simulink library "lib_lowphy"  (R2023b)
settings: Solver=VariableStepAuto  StartTime=0.0  StopTime=10.0  RelTol=1e-3
undefined symbols (not defined in the file or in its folder): AdvDSPBChannelOutDisplay, AdvDSPBDMemDisplay, AdvDSPBInDisplay, AdvDSPBOutDisplay, dpoly, dspba, dspba_ChannelInVis, dspba_ChannelOutVis, dspba_internal_get_channel_ports, evalAionMaskParam, fft_tb_in, ifft_tb_in, latency, latencyCorrection, max_FFTStages, max_NSubcarriers, primtype, UseDontCare, value
libraries: DSPBAPrim x637, DSPBAControl x55, $bdroot x16, DSPBAModelBus x12, DSPBAUtilities x6, DSPBABase x5, DSPBAWaveformSynth x4, DspbAdvFftLibrary x3, DSPBAVectorUtil x2, DspbAdvVfftPrefix x1
(part 3 of 9)

== system lib_lowphy/PhaseCompensation_lite/SOP_EOP_gen ==
  vin : Inport
  chin : Inport  Port=2
  din : Inport  Port=3
  eAxC_in : Inport  Port=4
  And : DSPBAPrim/And  primtype=and  nInputs=2  nOutputs=1  omode=Inherit via internal rule  otype=sfix(16)  scale=2^-15  rndmethod=Unbiased  factor=1  satmethod=Symmetric  shift_vec=[0 1 2 -1]  value=0  inPortNames=[' '; ' '; ' '; ' '; ' '; ' '; ' '; ' '; ' '; ' '; ' '; ' '; ' '; ' '; ' '; ' '; ]  outPortNames=[' ']  dspbaimage=dspba_prim.svg  text=fprintf('&');  style=Optimised  visibilities=8+2  version=20211007
  And1 : DSPBAPrim/And  primtype=and  nInputs=2  nOutputs=1  omode=Inherit via internal rule  otype=sfix(16)  scale=2^-15  rndmethod=Unbiased  factor=1  satmethod=Symmetric  shift_vec=[0 1 2 -1]  value=0  inPortNames=[' '; ' '; ' '; ' '; ' '; ' '; ' '; ' '; ' '; ' '; ' '; ' '; ' '; ' '; ' '; ' '; ]  outPortNames=[' ']  dspbaimage=dspba_prim.svg  text=fprintf('&');  style=Optimised  visibilities=8+2  version=20211007
  CmpEQ : DSPBAPrim/CmpEQ  primtype=cmpeq  nInputs=2  nOutputs=1  omode=boolean  otype=sfix(16)  scale=2^-15  rndmethod=Unbiased  factor=1  satmethod=Symmetric  shift_vec=[0 1 2 -1]  value=0  inPortNames=[' '; ' ';]  outPortNames=[' ']  dspbaimage=dspba_prim.svg  text=fprintf('==');  style=Optimised  visibilities=0  advOptions=[]  version=20211007
  CmpEQ1 : DSPBAPrim/CmpEQ  primtype=cmpeq  nInputs=2  nOutputs=1  omode=boolean  otype=sfix(16)  scale=2^-15  rndmethod=Unbiased  factor=1  satmethod=Symmetric  shift_vec=[0 1 2 -1]  value=0  inPortNames=[' '; ' ';]  outPortNames=[' ']  dspbaimage=dspba_prim.svg  text=fprintf('==');  style=Optimised  visibilities=0  advOptions=[]  version=20211007
  Const : DSPBAPrim/Const  primtype=const  nInputs=0  nOutputs=1  omode=Specify via dialog  otype=uint(8)  scale=2^0  rndmethod=Unbiased  factor=1  satmethod=Symmetric  shift_vec=[0 1 2 -1]  value=3  inPortNames=['+'; '+';]  outPortNames=[' ']  dspbaimage=dspba_prim.svg  text=fprintf('%s', num2str(value));  style=Optimised  visibilities=8 + 1024  floatPrecision=float32_m23  warnSaturation=on  version=20211007  SampleTime=inf
  Const1 : DSPBAPrim/Const  primtype=const  nInputs=0  nOutputs=1  omode=Specify via dialog  otype=uint(8)  scale=2^0  rndmethod=Unbiased  factor=1  satmethod=Symmetric  shift_vec=[0 1 2 -1]  value=0  inPortNames=['+'; '+';]  outPortNames=[' ']  dspbaimage=dspba_prim.svg  text=fprintf('%s', num2str(value));  style=Optimised  visibilities=8 + 1024  floatPrecision=float32_m23  warnSaturation=on  version=20211007  SampleTime=inf
  Rising_edge : Subsystem
      mask init:
      | fsmpaths
  SampleDelay{1..4} (4 alike) : DSPBAPrim/SampleDelay  primtype=sampdelay  nInputs=1  nOutputs=1  omode=Inherit via internal rule  otype=sfix(16)  scale=2^-15  rndmethod=Unbiased  factor=1  satmethod=Symmetric  shift_vec=[0 1 2 -1]  floatPrecision=float32_m23  value=1  inPortNames=[' '; ' ';]  outPortNames=[' ']  dspbaimage=dspba_prim.svg  text=dpoly(1, eye(1,value+1), 'z')  style=Optimised  visibilities=8 + 1024 + 2^17 + 2^18  flexible=off  slackgroup=0  augmented=3  version=20211007  advOptions=[]
  SynthesisInfo : DSPBAPrim/SynthesisInfo  primtype=synthinfo  nInputs=0  nOutputs=0  omode=Inherit via internal rule  otype=sfix(16)  scale=2^-15  rndmethod=Truncate  factor=1  satmethod=Symmetric  shift_vec=[0 1 2 -1]  value=99  inPortNames=[' '; ' ';]  outPortNames=[' ']  dspbaimage=dspba_prim_ctrl.jpg  text=fprintf('Style=%s', style);  style=Scheduled  visibilities=2^17+2^18+2^19+2^20+2^21+2^22+2^23+2^24  constraintPair=None  constraintRelation=>  constraintLimit=2  modelRefSign=+  modelRef=''  showSchedule=off  simulationMode=Use Global Value  resetMinimization=Conditional - On for ChannelIn/Out only  version=20220106
  channel_RXG1_in : DSPBAPrim/ChannelIn  primtype=channelin  nInputs=dspba_internal_get_channel_ports(gcb)  nOutputs=dspba_internal_get_channel_ports(gcb)  omode=Inherit via internal rule  otype=sfix(16)  scale=2^-15  rndmethod=Unbiased  factor=1  satmethod=Symmetric  shift_vec=[0 1 2 -1]  value=2  inPortNames=['v'; 'c'; '0'; '1'; '2'; '3'; '4'; '5'; '6'; '7'; '8'; '9'; 'A'; 'B'; 'D'; 'E'; 'F'; 'G'; 'H'; 'I'; 'J'; 'K'; 'L'; 'M'; 'N'; 'O'; 'P'; 'Q'; 'R'; 'S'; 'T'; 'U'; 'W'; 'X'; 'Y'; 'Z']  outPortNames=['v'; 'c'; '0'; '1'; '2'; '3'; '4'; '5'; '6'; '7'; '8'; '9'; 'A'; 'B'; 'D'; 'E'; 'F'; 'G'; 'H'; 'I'; 'J'; 'K'; 'L'; 'M'; 'N'; 'O'; 'P'; 'Q'; 'R'; 'S'; 'T'; 'U'; 'W'; 'X'; 'Y'; 'Z']  dspbaimage=dspba_prim_channel_tall.svg  text=fprintf('In');  style=Optimised  dataSignals=2  foldingEnabled=off  channels=1  sampleRate=200  packetBeginPresent=off  packetBeginEnabled=off  visibilities=dspba_ChannelInVis(gcb)  latencyCorrection=0  scheduleOrigin=on  version=20211214
  channel_RXG1_out : DSPBAPrim/ChannelOut  primtype=channelout  nInputs=dspba_internal_get_channel_ports(gcb)  nOutputs=dspba_internal_get_channel_ports(gcb)  omode=Inherit via internal rule  otype=sfix(16)  scale=2^-15  rndmethod=Unbiased  factor=1  satmethod=Symmetric  shift_vec=[0 1 2 -1]  value=6  inPortNames=['v'; 'c'; '0'; '1'; '2'; '3'; '4'; '5'; '6'; '7'; '8'; '9'; 'A'; 'B'; 'D'; 'E'; 'F'; 'G'; 'H'; 'I'; 'J'; 'K'; 'L'; 'M'; 'N'; 'O'; 'P'; 'Q'; 'R'; 'S'; 'T'; 'U'; 'W'; 'X'; 'Y'; 'Z']  outPortNames=['v'; 'c'; '0'; '1'; '2'; '3'; '4'; '5'; '6'; '7'; '8'; '9'; 'A'; 'B'; 'D'; 'E'; 'F'; 'G'; 'H'; 'I'; 'J'; 'K'; 'L'; 'M'; 'N'; 'O'; 'P'; 'Q'; 'R'; 'S'; 'T'; 'U'; 'W'; 'X'; 'Y'; 'Z']  dspbaimage=dspba_prim_channel_tall.svg  text=fprintf('Out%s', AdvDSPBChannelOutDisplay(latency));  style=Optimised  dataSignals=6  foldingEnabled=off  channels=1  sampleRate=200  packetBeginPresent=off  packetBeginEnabled=off  visibilities=dspba_ChannelOutVis(gcb)  latency=8  latencyCorrection=0  version=20211214
  falling_edge : Subsystem
      mask init:
      | fsmpaths
  vout : Outport
  chout : Outport  Port=2
  dout : Outport  Port=3
  eAxC_out : Outport  Port=4
  eop_eAxC : Outport  Port=5
  eop_sym : Outport  Port=6
  sop_eAxC : Outport  Port=7
  sop_sym : Outport  Port=8
  wires:
  falling_edge/1(falling_edge) -> And/1, channel_RXG1_out/5
  channel_RXG1_out/4 -> eAxC_out/1
  channel_RXG1_in/1 -> falling_edge/1(in), SampleDelay2/1
  channel_RXG1_in/4 -> CmpEQ/2, SampleDelay4/1
  channel_RXG1_out/1 -> vout/1
  channel_RXG1_out/5 -> eop_eAxC/1
  channel_RXG1_out/6 -> eop_sym/1
  vin/1 -> channel_RXG1_in/1
  channel_RXG1_in/2 -> SampleDelay1/1
  eAxC_in/1 -> channel_RXG1_in/4
  chin/1 -> channel_RXG1_in/2
  din/1 -> channel_RXG1_in/3
  channel_RXG1_in/3 -> SampleDelay3/1
  channel_RXG1_out/2 -> chout/1
  Const/1 -> CmpEQ/1
  And/1 -> channel_RXG1_out/6
  channel_RXG1_out/3 -> dout/1
  CmpEQ/1 -> And/2
  SampleDelay2/1 -> Rising_edge/1(in), channel_RXG1_out/1
  SampleDelay1/1 -> channel_RXG1_out/2
  SampleDelay3/1 -> channel_RXG1_out/3
  channel_RXG1_out/7 -> sop_eAxC/1
  channel_RXG1_out/8 -> sop_sym/1
  Const1/1 -> CmpEQ1/1
  SampleDelay4/1 -> CmpEQ1/2, channel_RXG1_out/4
  Rising_edge/1(rising_edge) -> And1/1, channel_RXG1_out/7
  CmpEQ1/1 -> And1/2
  And1/1 -> channel_RXG1_out/8

== system lib_lowphy/iFFT_B2S/B2S ==
  v_in : Inport
  c_in : Inport  Port=2
  q_in : Inport  Port=3
  sizein : Inport  Port=4
  cplen : Inport  Port=5
  nprb : Inport  Port=6
  B2S_Inst : Subsystem
  vout1 : Outport
  cout1 : Outport  Port=2
  dout1 : Outport  Port=3
  wires:
  cplen/1 -> B2S_Inst/5(cplen)
  c_in/1 -> B2S_Inst/2(chin)
  q_in/1 -> B2S_Inst/3(din)
  sizein/1 -> B2S_Inst/4(FFTSize)
  v_in/1 -> B2S_Inst/1(vin)
  B2S_Inst/1(vout) -> vout1/1
  B2S_Inst/2(cout) -> cout1/1
  B2S_Inst/3(q) -> dout1/1
  nprb/1 -> B2S_Inst/6(nprb)

== system lib_lowphy/iFFT_B2S/IFFT ==
  note: VIFFT :4 AxCs of 100 MHz
  data1 : Inport
  valid1 : Inport  Port=2
  channel1 : Inport  Port=3
  size1 : Inport  Port=4
  cplen1 : Inport  Port=5
  nsc1 : Inport  Port=6
  ifft_gain_re_l1 : Inport  Port=7
  ifft_gain_im_l1 : Inport  Port=8
  ifft_shift_l1 : Inport  Port=9
  ifft_mux_const_l1 : Inport  Port=10
  muxsel_l1 : Inport  Port=11
  DC_SC_EN : Inport  Port=12
  ripple_comp_en : Inport  Port=13
  rc_bw_sel : Inport  Port=14
  time_in : Inport  Port=15
  Input_signal_latch : Subsystem
  VIFFT : Subsystem
  vout1 : Outport
  cout1 : Outport  Port=2
  dout1 : Outport  Port=3
  sizeout1 : Outport  Port=4
  cpout1 : Outport  Port=5
  nprb : Outport  Port=6
  fd_data_v : Outport  Port=7
  fd_data_c : Outport  Port=8
  fd_data_q : Outport  Port=9
  fd_time_out : Outport  Port=10
  wires:
  VIFFT/1(dout) -> dout1/1
  VIFFT/5(cplen_Out) -> cpout1/1
  VIFFT/3(cout) -> cout1/1
  valid1/1 -> Input_signal_latch/1(valid)
  Input_signal_latch/5(q_nprb) -> VIFFT/6(nsc)
  Input_signal_latch/2(qchannel) -> VIFFT/3(channel)
  ifft_mux_const_l1/1 -> Input_signal_latch/11(ifft_mux_const_data)
  VIFFT/2(vout) -> vout1/1
  Input_signal_latch/4(qfftsize) -> VIFFT/4(size)
  Input_signal_latch/9(qf_ift_gain_imag) -> VIFFT/8(ifft_gain_im)
  cplen1/1 -> Input_signal_latch/6(cplen)
  data1/1 -> Input_signal_latch/3(data)
  Input_signal_latch/6(qcplen) -> VIFFT/5(cplen)
  Input_signal_latch/7(q_dc_sc_en) -> VIFFT/12(DC_SC_EN)
  Input_signal_latch/3(qdata) -> VIFFT/1(data)
  ifft_gain_im_l1/1 -> Input_signal_latch/9(ifftgain_imag)
  Input_signal_latch/11(q_ifft_mux_const_data) -> VIFFT/10(ifft_mux_const)
  VIFFT/4(sizeout) -> sizeout1/1
  Input_signal_latch/10(q_ifftshift) -> VIFFT/9(ifft_shift)
  Input_signal_latch/12(q_muxsel) -> VIFFT/11(muxsel)
  Input_signal_latch/8(qfft_gain_real) -> VIFFT/7(ifft_gain_re)
  Input_signal_latch/1(qvalid) -> VIFFT/2(valid)
  DC_SC_EN/1 -> Input_signal_latch/7(DC_SC_EN1)
  nsc1/1 -> Input_signal_latch/5(NSubCarr)
  muxsel_l1/1 -> Input_signal_latch/12(muxsel)
  ifft_shift_l1/1 -> Input_signal_latch/10(ifftshift)
  ifft_gain_re_l1/1 -> Input_signal_latch/8(iftgain_real)
  size1/1 -> Input_signal_latch/4(FFTSize)
  channel1/1 -> Input_signal_latch/2(ch)
  VIFFT/6(nprb) -> nprb/1
  ripple_comp_en/1 -> VIFFT/13(ripple_comp_en)
  rc_bw_sel/1 -> VIFFT/14(rc_bw_sel)
  VIFFT/7(fd_data_v) -> fd_data_v/1
  VIFFT/8(fd_data_c) -> fd_data_c/1
  VIFFT/9(fd_data_q) -> fd_data_q/1
  time_in/1 -> Input_signal_latch/13(time_in)
  Input_signal_latch/13(time_out) -> VIFFT/15(time_in)
  VIFFT/10(fd_time_out) -> fd_time_out/1

== system lib_lowphy/FFT_S2B/CPRemoval/Incr_Symbol_out_val ==
  dv : Inport
  Sym_counter_meta_data : Subsystem
  Sym_out_meta : Outport
  wires:
  Sym_counter_meta_data/1(Sym_out_meta) -> Sym_out_meta/1
  dv/1 -> Sym_counter_meta_data/1(Data_write_valid)

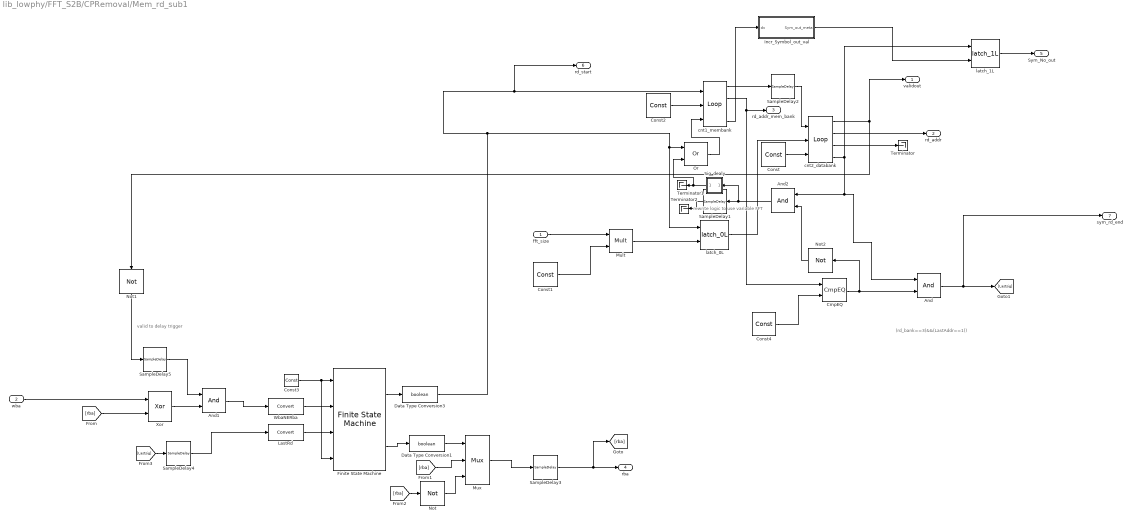
== system lib_lowphy/FFT_S2B/CPRemoval/Mem_rd_sub1 ==
  note: rewrite logic to use variable FFT
  note: (rd_bank==3)&&(LastAddr==1))
  note: valid to delay trigger
  fft_size : Inport
  wba : Inport  Port=2
  And : DSPBAPrim/And  primtype=and  nInputs=2  nOutputs=1  omode=Inherit via internal rule  otype=sfix(16)  scale=2^-15  rndmethod=Unbiased  factor=1  satmethod=Symmetric  shift_vec=[0 1 2 -1]  value=0  inPortNames=[' '; ' '; ' '; ' '; ' '; ' '; ' '; ' '; ' '; ' '; ' '; ' '; ' '; ' '; ' '; ' '; ]  outPortNames=[' ']  dspbaimage=dspba_prim.svg  text=fprintf('&');  style=Optimised  visibilities=8+2  version=20211007
  And1 : DSPBAPrim/And  primtype=and  nInputs=2  nOutputs=1  omode=Inherit via internal rule  otype=sfix(16)  scale=2^-15  rndmethod=Unbiased  factor=1  satmethod=Symmetric  shift_vec=[0 1 2 -1]  value=0  inPortNames=[' '; ' '; ' '; ' '; ' '; ' '; ' '; ' '; ' '; ' '; ' '; ' '; ' '; ' '; ' '; ' '; ]  outPortNames=[' ']  dspbaimage=dspba_prim.svg  text=fprintf('&');  style=Optimised  visibilities=8+2  version=20211007
  And2 : DSPBAPrim/And  primtype=and  nInputs=2  nOutputs=1  omode=Inherit via internal rule  otype=sfix(16)  scale=2^-15  rndmethod=Unbiased  factor=1  satmethod=Symmetric  shift_vec=[0 1 2 -1]  value=0  inPortNames=[' '; ' '; ' '; ' '; ' '; ' '; ' '; ' '; ' '; ' '; ' '; ' '; ' '; ' '; ' '; ' '; ]  outPortNames=[' ']  dspbaimage=dspba_prim.svg  text=fprintf('&');  style=Optimised  visibilities=8+2  version=20211007
  CmpEQ : DSPBAPrim/CmpEQ  primtype=cmpeq  nInputs=2  nOutputs=1  omode=boolean  otype=sfix(16)  scale=2^-15  rndmethod=Unbiased  factor=1  satmethod=Symmetric  shift_vec=[0 1 2 -1]  value=0  inPortNames=[' '; ' ';]  outPortNames=[' ']  dspbaimage=dspba_prim.svg  text=fprintf('==');  style=Optimised  visibilities=0  advOptions=[]  version=20211007
  Const : DSPBAPrim/Const  primtype=const  nInputs=0  nOutputs=1  omode=boolean  otype=sfix(16)  scale=2^-15  rndmethod=Unbiased  factor=1  satmethod=Symmetric  shift_vec=[0 1 2 -1]  value=1  inPortNames=['+'; '+';]  outPortNames=[' ']  dspbaimage=dspba_prim.svg  text=fprintf('%s', num2str(value));  style=Optimised  visibilities=8 + 1024  floatPrecision=float32_m23  warnSaturation=on  version=20211007  SampleTime=inf
  Const1 : DSPBAPrim/Const  primtype=const  nInputs=0  nOutputs=1  omode=Specify via dialog  otype=fixdt(0,3,0)  scale=0  rndmethod=Unbiased  factor=1  satmethod=Symmetric  shift_vec=[0 1 2 -1]  value=1  inPortNames=['+'; '+';]  outPortNames=[' ']  dspbaimage=dspba_prim.svg  text=fprintf('%s', num2str(value));  style=Optimised  visibilities=8 + 1024  floatPrecision=float32_m23  warnSaturation=on  version=20211007  SampleTime=inf
  Const2 : DSPBAPrim/Const  primtype=const  nInputs=0  nOutputs=1  omode=Specify via dialog  otype=fixdt(0,3,0)  scale=0  rndmethod=Unbiased  factor=1  satmethod=Symmetric  shift_vec=[0 1 2 -1]  value=4  inPortNames=['+'; '+';]  outPortNames=[' ']  dspbaimage=dspba_prim.svg  text=fprintf('%s', num2str(value));  style=Optimised  visibilities=8 + 1024  floatPrecision=float32_m23  warnSaturation=on  version=20211007  SampleTime=inf
  Const3 : DSPBAPrim/Const  primtype=const  nInputs=0  nOutputs=1  omode=Specify via dialog  otype=ufix(1)  scale=1  rndmethod=Unbiased  factor=1  satmethod=Symmetric  shift_vec=[0 1 2 -1]  value=1  inPortNames=['+'; '+';]  outPortNames=[' ']  dspbaimage=dspba_prim.svg  text=fprintf('%s', num2str(value));  style=Optimised  visibilities=8 + 1024  floatPrecision=float32_m23  warnSaturation=on  version=20211007  SampleTime=inf
  Const4 : DSPBAPrim/Const  primtype=const  nInputs=0  nOutputs=1  omode=Specify via dialog  otype=fixdt(0,3,0)  scale=0  rndmethod=Unbiased  factor=1  satmethod=Symmetric  shift_vec=[0 1 2 -1]  value=3  inPortNames=['+'; '+';]  outPortNames=[' ']  dspbaimage=dspba_prim.svg  text=fprintf('%s', num2str(value));  style=Optimised  visibilities=8 + 1024  floatPrecision=float32_m23  warnSaturation=on  version=20211007  SampleTime=inf
  Data Type Conversion1 : DataTypeConversion  OutDataTypeStr=boolean  SaturateOnIntegerOverflow=off  RndMeth=Floor
  Data Type Conversion3 : DataTypeConversion  OutDataTypeStr=boolean  SaturateOnIntegerOverflow=off  RndMeth=Floor
  Finite State Machine : DSPBAUtilities/Finite State Machine  desc_file=demo_fsm_control_read_s2b.fsm  latency=0  simulationMode=Bit And Cycle Accurate  finiteStateMachine=on
  Incr_Symbol_out_val : Subsystem
  LastRd : DataTypeConversion  SaturateOnIntegerOverflow=off  RndMeth=Floor
  Mult : DSPBAPrim/Mult  primtype=mult  nInputs=2  nOutputs=1  omode=Inherit via internal rule  otype=sfix(16)  scale=2^-15  rndmethod=Unbiased  factor=1  satmethod=Symmetric  shift_vec=[0 1 2 -1]  value=0  inPortNames=[' '; ' ';]  outPortNames=[' ']  dspbaimage=dspba_prim.svg  text=fprintf('X');  style=Optimised  visibilities=8+2^18+2^19  floatPrecision=float32_m23  floatRounding=correct  advOptions=[]  version=20211007
  Mux : DSPBAPrim/Mux  primtype=mux  nInputs=evalAionMaskParam(gcb,'value',1)+1  nOutputs=1  omode=Inherit via internal rule  otype=sfix(16)  scale=2^-15  rndmethod=Unbiased  factor=1  satmethod=Symmetric  shift_vec=[0 1 2 -1]  value=2  inPortNames=['s '; 'd0'; 'd1'; 'd2'; 'd3'; 'd4'; 'd5'; 'd6'; 'd7'; 'd8'; 'd9';]  outPortNames=[' ']  dspbaimage=dspba_prim_tall.svg  text=fprintf('%s', primtype);  style=Optimised  visibilities=1032  version=20211007
  Not : DSPBAPrim/Not  primtype=not  nInputs=1  nOutputs=1  omode=Inherit via internal rule  otype=sfix(16)  scale=2^-15  rndmethod=Unbiased  factor=1  satmethod=Symmetric  shift_vec=[0 1 2 -1]  value=0  inPortNames=[' '; ' ';]  outPortNames=[' ']  dspbaimage=dspba_prim.svg  text=fprintf('~');  style=Optimised  visibilities=8  version=20211007
  Not1 : DSPBAPrim/Not  primtype=not  nInputs=1  nOutputs=1  omode=Inherit via internal rule  otype=sfix(16)  scale=2^-15  rndmethod=Unbiased  factor=1  satmethod=Symmetric  shift_vec=[0 1 2 -1]  value=0  inPortNames=[' '; ' ';]  outPortNames=[' ']  dspbaimage=dspba_prim.svg  text=fprintf('~');  style=Optimised  visibilities=8  version=20211007
  Not2 : DSPBAPrim/Not  primtype=not  nInputs=1  nOutputs=1  omode=Inherit via internal rule  otype=sfix(16)  scale=2^-15  rndmethod=Unbiased  factor=1  satmethod=Symmetric  shift_vec=[0 1 2 -1]  value=0  inPortNames=[' '; ' ';]  outPortNames=[' ']  dspbaimage=dspba_prim.svg  text=fprintf('~');  style=Optimised  visibilities=8  version=20211007
  Or : DSPBAPrim/Or  primtype=or  nInputs=2  nOutputs=1  omode=Inherit via internal rule  otype=sfix(16)  scale=2^-15  rndmethod=Unbiased  factor=1  satmethod=Symmetric  shift_vec=[0 1 2 -1]  value=0  inPortNames=[' '; ' '; ' '; ' '; ' '; ' '; ' '; ' '; ' '; ' '; ' '; ' '; ' '; ' '; ' '; ' '; ]  outPortNames=[' ']  dspbaimage=dspba_prim.svg  text=fprintf('|');  style=Optimised  visibilities=8+2  version=20211007
  SampleDelay1 : DSPBAPrim/SampleDelay  primtype=sampdelay  nInputs=1  nOutputs=1  omode=Inherit via internal rule  otype=sfix(16)  scale=2^-15  rndmethod=Unbiased  factor=1  satmethod=Symmetric  shift_vec=[0 1 2 -1]  floatPrecision=float32_m23  value=288  inPortNames=[' '; ' ';]  outPortNames=[' ']  dspbaimage=dspba_prim.svg  text=dpoly(1, eye(1,value+1), 'z')  style=Optimised  visibilities=8 + 1024 + 2^17 + 2^18  flexible=off  slackgroup=0  augmented=0  version=20211007  advOptions=[]
  SampleDelay2 : DSPBAPrim/SampleDelay  primtype=sampdelay  nInputs=1  nOutputs=1  omode=Inherit via internal rule  otype=sfix(16)  scale=2^-15  rndmethod=Unbiased  factor=1  satmethod=Symmetric  shift_vec=[0 1 2 -1]  floatPrecision=float32_m23  value=1  inPortNames=[' '; ' ';]  outPortNames=[' ']  dspbaimage=dspba_prim.svg  text=dpoly(1, eye(1,value+1), 'z')  style=Optimised  visibilities=8 + 1024 + 2^17 + 2^18  flexible=on  slackgroup=0  augmented=3  version=20211007  advOptions=[]
  SampleDelay3 : DSPBAPrim/SampleDelay  primtype=sampdelay  nInputs=1  nOutputs=1  omode=boolean  otype=sfix(16)  scale=2^-15  rndmethod=Unbiased  factor=1  satmethod=Symmetric  shift_vec=[0 1 2 -1]  floatPrecision=float32_m23  value=1  inPortNames=[' '; ' ';]  outPortNames=[' ']  dspbaimage=dspba_prim.svg  text=dpoly(1, eye(1,value+1), 'z')  style=Optimised  visibilities=8 + 1024 + 2^17 + 2^18  flexible=off  slackgroup=0  augmented=0  version=20211007  advOptions=[]
  SampleDelay4 : DSPBAPrim/SampleDelay  primtype=sampdelay  nInputs=1  nOutputs=1  omode=Inherit via internal rule  otype=sfix(16)  scale=2^-15  rndmethod=Unbiased  factor=1  satmethod=Symmetric  shift_vec=[0 1 2 -1]  floatPrecision=float32_m23  value=1  inPortNames=[' '; ' ';]  outPortNames=[' ']  dspbaimage=dspba_prim.svg  text=dpoly(1, eye(1,value+1), 'z')  style=Optimised  visibilities=8 + 1024 + 2^17 + 2^18  flexible=off  slackgroup=0  augmented=0  version=20211007  advOptions=[]
  SampleDelay5 : DSPBAPrim/SampleDelay  primtype=sampdelay  nInputs=1  nOutputs=1  omode=Inherit via internal rule  otype=sfix(16)  scale=2^-15  rndmethod=Unbiased  factor=1  satmethod=Symmetric  shift_vec=[0 1 2 -1]  floatPrecision=float32_m23  value=10  inPortNames=[' '; ' ';]  outPortNames=[' ']  dspbaimage=dspba_prim.svg  text=dpoly(1, eye(1,value+1), 'z')  style=Optimised  visibilities=8 + 1024 + 2^17 + 2^18  flexible=off  slackgroup=0  augmented=0  version=20211007  advOptions=[]
  Sig_dealy : Subsystem
  Terminator : Terminator
  Terminator1 : Terminator
  Terminator2 : Terminator
  WbaNERba : DataTypeConversion  SaturateOnIntegerOverflow=off  RndMeth=Floor
  Xor : DSPBAPrim/Xor  primtype=xor  nInputs=2  nOutputs=1  omode=boolean  otype=sfix(16)  scale=2^-15  rndmethod=Unbiased  factor=1  satmethod=Symmetric  shift_vec=[0 1 2 -1]  value=0  inPortNames=[' '; ' '; ' '; ' '; ' '; ' '; ' '; ' '; ' '; ' '; ' '; ' '; ' '; ' '; ' '; ' '; ]  outPortNames=[' ']  dspbaimage=dspba_prim.svg  text=fprintf('^');  style=Optimised  visibilities=8+2  version=20211007
  cnt1_membank : DSPBAPrim/Loop  primtype=loop  nInputs=3  nOutputs=4  omode=Inherit via internal rule  otype=sfix(16)  scale=2^-15  rndmethod=Unbiased  factor=1  satmethod=Symmetric  shift_vec=[0 1 2 -1]  value=[zeros(16, 1)]  inPortNames=['g'; 'c'; 'e']  outPortNames=['v'; 'q'; 'f'; 'l']  dspbaimage=dspba_prim_tall.svg  text=fprintf('loop');  style=Optimised  visibilities=0  version=20211007
  cnt2_databank : DSPBAPrim/Loop  primtype=loop  nInputs=3  nOutputs=4  omode=Inherit via internal rule  otype=sfix(16)  scale=2^-15  rndmethod=Unbiased  factor=1  satmethod=Symmetric  shift_vec=[0 1 2 -1]  value=[zeros(16, 1)]  inPortNames=['g'; 'c'; 'e']  outPortNames=['v'; 'q'; 'f'; 'l']  dspbaimage=dspba_prim_tall.svg  text=fprintf('loop');  style=Optimised  visibilities=0  version=20211007
  latch_0L : DSPBAControl/latch_0L
  latch_1L : DSPBAControl/latch_1L
  validout : Outport
  rd_addr : Outport  Port=2
  rd_addr_mem_bank : Outport  Port=3
  rba : Outport  Port=4
  Sym_No_out : Outport  Port=5
  rd_start : Outport  Port=6
  sym_rd_end : Outport  Port=7
  wires:
  cnt2_databank/2 -> rd_addr/1
  cnt2_databank/1 -> validout/1, Not1/1
  cnt2_databank/3 -> Terminator/1
  Data Type Conversion3/1 -> rd_start/1, cnt1_membank/1, latch_0L/1, Or/1
  latch_0L/1 -> cnt2_databank/2
  Const/1 -> cnt2_databank/3
  Mult/1 -> latch_0L/2
  fft_size/1 -> Mult/1
  Const1/1 -> Mult/2
  Const2/1 -> cnt1_membank/2
  cnt1_membank/1 -> SampleDelay2/1
  cnt1_membank/2 -> CmpEQ/1, rd_addr_mem_bank/1
  SampleDelay2/1 -> cnt2_databank/1
  Or/1 -> cnt1_membank/3
  Const3/1 -> Finite State Machine/4, Finite State Machine/1
  [Lastsig] -> SampleDelay4/1
  Finite State Machine/1 -> Data Type Conversion3/1
  LastRd/1 -> Finite State Machine/3
  WbaNERba/1 -> Finite State Machine/2
  wba/1 -> Xor/1
  SampleDelay3/1 -> [rba], rba/1
  Mux/1 -> SampleDelay3/1
  [rba] -> Xor/2
  [rba] -> Mux/2
  Not/1 -> Mux/3
  [rba] -> Not/1
  Const4/1 -> CmpEQ/2
  CmpEQ/1 -> And/2, Not2/1
  And/1 -> sym_rd_end/1, [Lastsig]
  SampleDelay4/1 -> LastRd/1
  Data Type Conversion1/1 -> Mux/1
  Finite State Machine/2 -> Data Type Conversion1/1
  And1/1 -> WbaNERba/1
  Xor/1 -> And1/2
  SampleDelay5/1 -> And1/1
  Not1/1 -> SampleDelay5/1
  cnt2_databank/4 -> latch_1L/1, And2/1, And/1
  And2/1 -> Sig_dealy/1(In1), SampleDelay1/1
  Not2/1 -> And2/2
  Sig_dealy/1(Out1) -> Or/2, Terminator1/1
  cnt1_membank/4 -> Incr_Symbol_out_val/1(dv)
  latch_1L/1 -> Sym_No_out/1
  Incr_Symbol_out_val/1(Sym_out_meta) -> latch_1L/2
  SampleDelay1/1 -> Terminator2/1

== system lib_lowphy/FFT_S2B/CPRemoval/Mem_wr_subsystem ==
  valid : Inport
  CPlen : Inport  Port=2
  FFTlen : Inport  Port=3
  NumAxc : Inport  Port=4
  Const : DSPBAPrim/Const  primtype=const  nInputs=0  nOutputs=1  omode=boolean  otype=sfix(16)  scale=2^-15  rndmethod=Unbiased  factor=1  satmethod=Symmetric  shift_vec=[0 1 2 -1]  value=1  inPortNames=['+'; '+';]  outPortNames=[' ']  dspbaimage=dspba_prim.svg  text=fprintf('%s', num2str(value));  style=Optimised  visibilities=8 + 1024  floatPrecision=float32_m23  warnSaturation=on  version=20211007  SampleTime=inf
  Const1 : DSPBAPrim/Const  primtype=const  nInputs=0  nOutputs=1  omode=boolean  otype=sfix(16)  scale=2^-15  rndmethod=Unbiased  factor=1  satmethod=Symmetric  shift_vec=[0 1 2 -1]  value=1  inPortNames=['+'; '+';]  outPortNames=[' ']  dspbaimage=dspba_prim.svg  text=fprintf('%s', num2str(value));  style=Optimised  visibilities=8 + 1024  floatPrecision=float32_m23  warnSaturation=on  version=20211007  SampleTime=inf
  Const2 : DSPBAPrim/Const  primtype=const  nInputs=0  nOutputs=1  omode=Specify via dialog  otype=ufix(1)  scale=1  rndmethod=Unbiased  factor=1  satmethod=Symmetric  shift_vec=[0 1 2 -1]  value=1  inPortNames=['+'; '+';]  outPortNames=[' ']  dspbaimage=dspba_prim.svg  text=fprintf('%s', num2str(value));  style=Optimised  visibilities=8 + 1024  floatPrecision=float32_m23  warnSaturation=on  version=20211007  SampleTime=inf
  Data Type Conversion : DataTypeConversion  SaturateOnIntegerOverflow=off  RndMeth=Floor
  Data Type Conversion1 : DataTypeConversion  OutDataTypeStr=boolean  SaturateOnIntegerOverflow=off  RndMeth=Floor
  Data Type Conversion2 : DataTypeConversion  OutDataTypeStr=boolean  SaturateOnIntegerOverflow=off  RndMeth=Floor
  Data Type Conversion3 : DataTypeConversion  OutDataTypeStr=boolean  SaturateOnIntegerOverflow=off  RndMeth=Floor
  Finite State Machine : DSPBAUtilities/Finite State Machine  desc_file=demo_fsm_control.fsm  latency=0  simulationMode=Bit And Cycle Accurate  finiteStateMachine=on
  LShift : DSPBAPrim/LShift  primtype=lshift  nInputs=2  nOutputs=1  omode=Specify via dialog  otype=fixdt(0,12,0)  scale=0  rndmethod=Unbiased  factor=1  satmethod=Symmetric  shift_vec=[0 1 2 -1]  value=0  inPortNames=['a'; 'b';]  outPortNames=[' ']  dspbaimage=dspba_prim.svg  text=fprintf('a << b');  style=Optimised  visibilities=8  version=20211007
  LShift1 : DSPBAPrim/LShift  primtype=lshift  nInputs=2  nOutputs=1  omode=Specify via dialog  otype=fixdt(0,17,0)  scale=0  rndmethod=Unbiased  factor=1  satmethod=Symmetric  shift_vec=[0 1 2 -1]  value=0  inPortNames=['a'; 'b';]  outPortNames=[' ']  dspbaimage=dspba_prim.svg  text=fprintf('a << b');  style=Optimised  visibilities=8  version=20211007
  Lastsig_gen : Subsystem
  Lastsig_gen1 : $bdroot/FFT_S2B/CPRemoval/Mem_wr_subsystem/Lastsig_gen  SystemSampleTime=-1  VariantActivationTime=update diagram  AllowFlexibleInterface=on  Latency=0  AutoFrameSizeCalculation=off
  Mux : DSPBAPrim/Mux  primtype=mux  nInputs=evalAionMaskParam(gcb,'value',1)+1  nOutputs=1  omode=Inherit via internal rule  otype=sfix(16)  scale=2^-15  rndmethod=Unbiased  factor=1  satmethod=Symmetric  shift_vec=[0 1 2 -1]  value=2  inPortNames=['s '; 'd0'; 'd1'; 'd2'; 'd3'; 'd4'; 'd5'; 'd6'; 'd7'; 'd8'; 'd9';]  outPortNames=[' ']  dspbaimage=dspba_prim_tall.svg  text=fprintf('%s', primtype);  style=Optimised  visibilities=1032  version=20211007
  Not : DSPBAPrim/Not  primtype=not  nInputs=1  nOutputs=1  omode=Inherit via internal rule  otype=sfix(16)  scale=2^-15  rndmethod=Unbiased  factor=1  satmethod=Symmetric  shift_vec=[0 1 2 -1]  value=0  inPortNames=[' '; ' ';]  outPortNames=[' ']  dspbaimage=dspba_prim.svg  text=fprintf('~');  style=Optimised  visibilities=8  version=20211007
  SampleDelay3 : DSPBAPrim/SampleDelay  primtype=sampdelay  nInputs=1  nOutputs=1  omode=boolean  otype=sfix(16)  scale=2^-15  rndmethod=Unbiased  factor=1  satmethod=Symmetric  shift_vec=[0 1 2 -1]  floatPrecision=float32_m23  value=1  inPortNames=[' '; ' ';]  outPortNames=[' ']  dspbaimage=dspba_prim.svg  text=dpoly(1, eye(1,value+1), 'z')  style=Optimised  visibilities=8 + 1024 + 2^17 + 2^18  flexible=off  slackgroup=0  augmented=0  version=20211007  advOptions=[]
  Terminator{,1..5} (6 alike) : Terminator
  cmp1in : DataTypeConversion  SaturateOnIntegerOverflow=off  RndMeth=Floor
  cmpin2 : DataTypeConversion  SaturateOnIntegerOverflow=off  RndMeth=Floor
  cnt1_cpcnt : DSPBAPrim/Loop  primtype=loop  nInputs=3  nOutputs=4  omode=Inherit via internal rule  otype=sfix(16)  scale=2^-15  rndmethod=Unbiased  factor=1  satmethod=Symmetric  shift_vec=[0 1 2 -1]  value=[zeros(16, 1)]  inPortNames=['g'; 'c'; 'e']  outPortNames=['v'; 'q'; 'f'; 'l']  dspbaimage=dspba_prim_tall.svg  text=fprintf('loop');  style=Optimised  visibilities=0  version=20211007
  cnt2_datalen : DSPBAPrim/Loop  primtype=loop  nInputs=3  nOutputs=4  omode=Inherit via internal rule  otype=sfix(16)  scale=2^-15  rndmethod=Unbiased  factor=1  satmethod=Symmetric  shift_vec=[0 1 2 -1]  value=[zeros(16, 1)]  inPortNames=['g'; 'c'; 'e']  outPortNames=['v'; 'q'; 'f'; 'l']  dspbaimage=dspba_prim_tall.svg  text=fprintf('loop');  style=Optimised  visibilities=0  version=20211007
  latch_0L : DSPBAControl/latch_0L
  latch_0L1 : DSPBAControl/latch_0L
  validout : Outport
  Wr_addr : Outport  Port=2
  wba : Outport  Port=3
  sym_wr_start : Outport  Port=4
  wires:
  Lastsig_gen1/1 -> Mux/1, cmpin2/1
  Const2/1 -> Finite State Machine/5, Finite State Machine/1
  Data Type Conversion3/1 -> latch_0L1/1, latch_0L/1
  SampleDelay3/1 -> Mux/2, Not/1, wba/1
  latch_0L/1 -> LShift/1
  Data Type Conversion2/1 -> Lastsig_gen1/2, cnt2_datalen/1
  Const/1 -> cnt1_cpcnt/3
  cnt1_cpcnt/3 -> Terminator3/1
  cnt2_datalen/1 -> Lastsig_gen1/4, validout/1
  LShift1/1 -> Lastsig_gen1/1, cnt2_datalen/2
  NumAxc/1 -> LShift/2, LShift1/2
  cmpin2/1 -> Finite State Machine/4
  CPlen/1 -> latch_0L/2
  LShift/1 -> Lastsig_gen/1(CountMax), cnt1_cpcnt/2
  cnt2_datalen/2 -> Lastsig_gen1/3, Wr_addr/1
  cnt1_cpcnt/2 -> Lastsig_gen/3(Runningcnt), Terminator2/1
  FFTlen/1 -> latch_0L1/2
  Finite State Machine/1 -> Data Type Conversion3/1
  Data Type Conversion/1 -> Finite State Machine/2
  Finite State Machine/3 -> Data Type Conversion1/1
  Finite State Machine/5 -> Terminator5/1
  Mux/1 -> SampleDelay3/1
  Not/1 -> Mux/3
  cmp1in/1 -> Finite State Machine/3
  Finite State Machine/2 -> Terminator4/1
  cnt1_cpcnt/1 -> Lastsig_gen/4(valid), Terminator1/1
  cnt2_datalen/3 -> Terminator/1
  Finite State Machine/4 -> Data Type Conversion2/1
  latch_0L1/1 -> LShift1/1
  Const1/1 -> cnt2_datalen/3
  Data Type Conversion1/1 -> Lastsig_gen/2(latch), cnt1_cpcnt/1
  valid/1 -> Data Type Conversion/1
  Lastsig_gen/1(Lastsig) -> cmp1in/1
  cnt1_cpcnt/4 -> sym_wr_start/1

== system lib_lowphy/FFT_S2B/CPRemoval/Nprb_fifo ==
  qv : Inport
  v : Inport  Port=2
  d : Inport  Port=3
  FIFO : DSPBAPrim/FIFO  primtype=fifo  nInputs=3  nOutputs=4  omode=Inherit via internal rule  otype=sfix(16)  scale=2^-15  rndmethod=Unbiased  factor=1  satmethod=Symmetric  shift_vec=[0 1 2 -1]  value=[16 16 16]  inPortNames=['w'; 'd'; 'r'; 'f']  outPortNames=['v'; 'q'; 't'; 'f']  dspbaimage=dspba_prim_tall.svg  text=fprintf('fifo');  style=Optimised  visibilities=263168  version=20211007  user_sclr=off
  RISING_EDGE1 : Subsystem
  RISING_EDGE3 : Subsystem
  Terminator1 : Terminator
  Terminator2 : Terminator
  Terminator3 : Terminator
  latch_0L3 : DSPBAControl/latch_0L
  q : Outport
  wires:
  FIFO/2 -> latch_0L3/2
  RISING_EDGE3/1(q) -> latch_0L3/1, FIFO/3
  FIFO/3 -> Terminator2/1
  latch_0L3/1 -> q/1
  d/1 -> FIFO/2
  FIFO/4 -> Terminator3/1
  v/1 -> RISING_EDGE1/1(d)
  qv/1 -> RISING_EDGE3/1(d)
  FIFO/1 -> Terminator1/1
  RISING_EDGE1/1(q) -> FIFO/1

== system lib_lowphy/FFT_S2B/CPRemoval/cp_len ==
  cplen : Inport
  sym_det : Inport  Port=2
  fftsize : Inport  Port=3
  CmpEQ : DSPBAPrim/CmpEQ  primtype=cmpeq  nInputs=2  nOutputs=1  omode=boolean  otype=sfix(16)  scale=2^-15  rndmethod=Unbiased  factor=1  satmethod=Symmetric  shift_vec=[0 1 2 -1]  value=0  inPortNames=[' '; ' ';]  outPortNames=[' ']  dspbaimage=dspba_prim.svg  text=fprintf('==');  style=Optimised  visibilities=0  advOptions=[]  version=20211007
  CmpEQ1 : DSPBAPrim/CmpEQ  primtype=cmpeq  nInputs=2  nOutputs=1  omode=boolean  otype=sfix(16)  scale=2^-15  rndmethod=Unbiased  factor=1  satmethod=Symmetric  shift_vec=[0 1 2 -1]  value=0  inPortNames=[' '; ' ';]  outPortNames=[' ']  dspbaimage=dspba_prim.svg  text=fprintf('==');  style=Optimised  visibilities=0  advOptions=[]  version=20211007
  Const1 : DSPBAPrim/Const  primtype=const  nInputs=0  nOutputs=1  omode=Inherit via internal rule  otype=sfix(16)  scale=2^-15  rndmethod=Unbiased  factor=1  satmethod=Symmetric  shift_vec=[0 1 2 -1]  value=0.9  inPortNames=['+'; '+';]  outPortNames=[' ']  dspbaimage=dspba_prim.svg  text=fprintf('%s', num2str(value));  style=Optimised  visibilities=8 + 1024  floatPrecision=float32_m23  warnSaturation=on  version=20211007  SampleTime=inf
  Const12 : DSPBAPrim/Const  primtype=const  nInputs=0  nOutputs=1  omode=Inherit via internal rule  otype=sfix(16)  scale=2^-15  rndmethod=Unbiased  factor=1  satmethod=Symmetric  shift_vec=[0 1 2 -1]  value=0.8181  inPortNames=['+'; '+';]  outPortNames=[' ']  dspbaimage=dspba_prim.svg  text=fprintf('%s', num2str(value));  style=Optimised  visibilities=8 + 1024  floatPrecision=float32_m23  warnSaturation=on  version=20211007  SampleTime=inf
  Const2 : DSPBAPrim/Const  primtype=const  nInputs=0  nOutputs=1  omode=Inherit via internal rule  otype=sfix(16)  scale=2^-15  rndmethod=Unbiased  factor=1  satmethod=Symmetric  shift_vec=[0 1 2 -1]  value=0  inPortNames=['+'; '+';]  outPortNames=[' ']  dspbaimage=dspba_prim.svg  text=fprintf('%s', num2str(value));  style=Optimised  visibilities=8 + 1024  floatPrecision=float32_m23  warnSaturation=on  version=20211007  SampleTime=inf
  Const3 : DSPBAPrim/Const  primtype=const  nInputs=0  nOutputs=1  omode=Inherit via internal rule  otype=sfix(16)  scale=2^-15  rndmethod=Unbiased  factor=1  satmethod=Symmetric  shift_vec=[0 1 2 -1]  value=12  inPortNames=['+'; '+';]  outPortNames=[' ']  dspbaimage=dspba_prim.svg  text=fprintf('%s', num2str(value));  style=Optimised  visibilities=8 + 1024  floatPrecision=float32_m23  warnSaturation=on  version=20211007  SampleTime=inf
  Convert : DSPBAPrim/Convert  primtype=convert  nInputs=1  nOutputs=1  omode=Specify via dialog  otype=ufix(11)  scale=2^-0  rndmethod=Biased  factor=1  satmethod=None  shift_vec=[0 1 2 -1]  value=round([0:255]/17)  inPortNames=[' '; ' ';]  outPortNames=[' '; 'c']  dspbaimage=dspba_prim_wide.svg  text=fprintf('convert');  style=Optimised  visibilities=8+64+256+2^17  clipdetect=off  floatPrecision=float32_m23  advOptions=[]  version=20211007
  Mult : DSPBAPrim/Mult  primtype=mult  nInputs=2  nOutputs=1  omode=Inherit via internal rule  otype=sfix(16)  scale=2^-15  rndmethod=Unbiased  factor=1  satmethod=Symmetric  shift_vec=[0 1 2 -1]  value=0  inPortNames=[' '; ' ';]  outPortNames=[' ']  dspbaimage=dspba_prim.svg  text=fprintf('X');  style=Optimised  visibilities=8+2^18+2^19  floatPrecision=float32_m23  floatRounding=correct  advOptions=[]  version=20211007
  Mux1 : DSPBAPrim/Mux  primtype=mux  nInputs=evalAionMaskParam(gcb,'value',1)+1  nOutputs=1  omode=Inherit via internal rule  otype=sfix(16)  scale=2^-15  rndmethod=Unbiased  factor=1  satmethod=Symmetric  shift_vec=[0 1 2 -1]  value=2  inPortNames=['s '; 'd0'; 'd1'; 'd2'; 'd3'; 'd4'; 'd5'; 'd6'; 'd7'; 'd8'; 'd9';]  outPortNames=[' ']  dspbaimage=dspba_prim_tall.svg  text=fprintf('%s', primtype);  style=Optimised  visibilities=1032  version=20211007
  Mux2 : DSPBAPrim/Mux  primtype=mux  nInputs=evalAionMaskParam(gcb,'value',1)+1  nOutputs=1  omode=Inherit via internal rule  otype=sfix(16)  scale=2^-15  rndmethod=Unbiased  factor=1  satmethod=Symmetric  shift_vec=[0 1 2 -1]  value=2  inPortNames=['s '; 'd0'; 'd1'; 'd2'; 'd3'; 'd4'; 'd5'; 'd6'; 'd7'; 'd8'; 'd9';]  outPortNames=[' ']  dspbaimage=dspba_prim_tall.svg  text=fprintf('%s', primtype);  style=Optimised  visibilities=1032  version=20211007
  cp_out : Outport
  wires:
  Convert/1 -> Mux2/2
  Mult/1 -> Convert/1
  cplen/1 -> Mult/1, Mux2/3
  Mux1/1 -> Mult/2
  Mux2/1 -> cp_out/1
  sym_det/1 -> CmpEQ/1
  CmpEQ/1 -> Mux2/1
  Const2/1 -> CmpEQ/2
  fftsize/1 -> CmpEQ1/1
  Const3/1 -> CmpEQ1/2
  Const12/1 -> Mux1/3
  CmpEQ1/1 -> Mux1/1
  Const1/1 -> Mux1/2

== system lib_lowphy/FFT_S2B/CPRemoval/fft_size_fifo ==
  qv : Inport
  v : Inport  Port=2
  d : Inport  Port=3
  FIFO : DSPBAPrim/FIFO  primtype=fifo  nInputs=3  nOutputs=4  omode=Inherit via internal rule  otype=sfix(16)  scale=2^-15  rndmethod=Unbiased  factor=1  satmethod=Symmetric  shift_vec=[0 1 2 -1]  value=[16 16 16]  inPortNames=['w'; 'd'; 'r'; 'f']  outPortNames=['v'; 'q'; 't'; 'f']  dspbaimage=dspba_prim_tall.svg  text=fprintf('fifo');  style=Optimised  visibilities=263168  version=20211007  user_sclr=off
  RISING_EDGE1 : Subsystem
  RISING_EDGE3 : Subsystem
  Terminator1 : Terminator
  Terminator2 : Terminator
  Terminator3 : Terminator
  latch_0L3 : DSPBAControl/latch_0L
  q : Outport
  wires:
  FIFO/2 -> latch_0L3/2
  RISING_EDGE3/1(q) -> latch_0L3/1, FIFO/3
  FIFO/3 -> Terminator2/1
  latch_0L3/1 -> q/1
  d/1 -> FIFO/2
  FIFO/4 -> Terminator3/1
  v/1 -> RISING_EDGE1/1(d)
  qv/1 -> RISING_EDGE3/1(d)
  FIFO/1 -> Terminator1/1
  RISING_EDGE1/1(q) -> FIFO/1

== system lib_lowphy/FFT_S2B/CPRemoval/sym_metadata_fffo ==
  qv : Inport
  v : Inport  Port=2
  d : Inport  Port=3
  FIFO : DSPBAPrim/FIFO  primtype=fifo  nInputs=3  nOutputs=4  omode=Inherit via internal rule  otype=sfix(16)  scale=2^-15  rndmethod=Unbiased  factor=1  satmethod=Symmetric  shift_vec=[0 1 2 -1]  value=[16 16 16]  inPortNames=['w'; 'd'; 'r'; 'f']  outPortNames=['v'; 'q'; 't'; 'f']  dspbaimage=dspba_prim_tall.svg  text=fprintf('fifo');  style=Optimised  visibilities=263168  version=20211007  user_sclr=off
  RISING_EDGE1 : Subsystem
  RISING_EDGE3 : Subsystem
  Terminator1 : Terminator
  Terminator2 : Terminator
  Terminator3 : Terminator
  q : Outport
  wires:
  RISING_EDGE3/1(q) -> FIFO/3
  FIFO/3 -> Terminator2/1
  FIFO/2 -> q/1
  d/1 -> FIFO/2
  FIFO/4 -> Terminator3/1
  v/1 -> RISING_EDGE1/1(d)
  qv/1 -> RISING_EDGE3/1(d)
  FIFO/1 -> Terminator1/1
  RISING_EDGE1/1(q) -> FIFO/1

== system lib_lowphy/FFT_S2B/CPRemoval/timeref_reg ==
  qv : Inport
  v : Inport  Port=2
  d : Inport  Port=3
  FIFO : DSPBAPrim/FIFO  primtype=fifo  nInputs=3  nOutputs=4  omode=Inherit via internal rule  otype=sfix(16)  scale=2^-15  rndmethod=Unbiased  factor=1  satmethod=Symmetric  shift_vec=[0 1 2 -1]  value=[16 16 16]  inPortNames=['w'; 'd'; 'r'; 'f']  outPortNames=['v'; 'q'; 't'; 'f']  dspbaimage=dspba_prim_tall.svg  text=fprintf('fifo');  style=Optimised  visibilities=263168  version=20211007  user_sclr=off
  RISING_EDGE1 : Subsystem
  RISING_EDGE3 : Subsystem
  Terminator1 : Terminator
  Terminator2 : Terminator
  Terminator3 : Terminator
  q : Outport
  wires:
  RISING_EDGE3/1(q) -> FIFO/3
  FIFO/3 -> Terminator2/1
  FIFO/2 -> q/1
  d/1 -> FIFO/2
  FIFO/4 -> Terminator3/1
  v/1 -> RISING_EDGE1/1(d)
  qv/1 -> RISING_EDGE3/1(d)
  FIFO/1 -> Terminator1/1
  RISING_EDGE1/1(q) -> FIFO/1

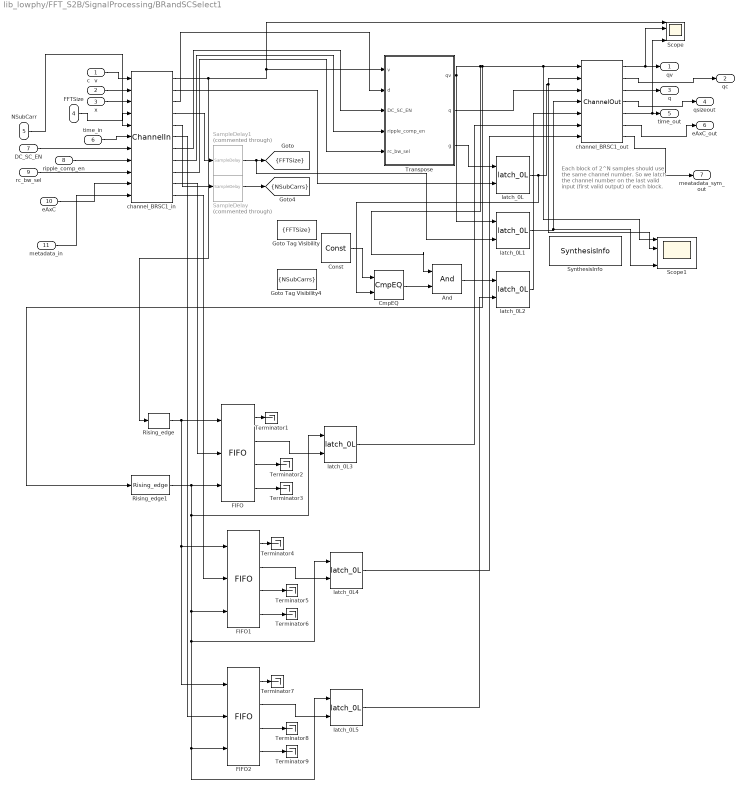
== system lib_lowphy/FFT_S2B/SignalProcessing/BRandSCSelect1 ==
  note: Each block of 2^N samples should
      |  use the same channel number.
      |
      | So we latch the channel number on
      |  the last valid input (first valid output)
      | of each block.
  v : Inport
  c : Inport  Port=2
  x : Inport  Port=3
  FFTSize : Inport  Port=4
  NSubCarr : Inport  Port=5
  time_in : Inport  Port=6
  DC_SC_EN : Inport  Port=7
  ripple_comp_en : Inport  Port=8
  rc_bw_sel : Inport  Port=9
  eAxC : Inport  Port=10
  metadata_in : Inport  Port=11
  And : DSPBAPrim/And  primtype=and  nInputs=2  nOutputs=1  omode=Inherit via internal rule  otype=sfix(16)  scale=2^-15  rndmethod=Unbiased  factor=1  satmethod=Symmetric  shift_vec=[0 1 2 -1]  value=0  inPortNames=[' '; ' '; ' '; ' '; ' '; ' '; ' '; ' '; ' '; ' '; ' '; ' '; ' '; ' '; ' '; ' '; ]  outPortNames=[' ']  dspbaimage=dspba_prim.svg  text=fprintf('&');  style=Optimised  visibilities=8+2  version=20211007
  CmpEQ : DSPBAPrim/CmpEQ  primtype=cmpeq  nInputs=2  nOutputs=1  omode=boolean  otype=sfix(16)  scale=2^-15  rndmethod=Unbiased  factor=1  satmethod=Symmetric  shift_vec=[0 1 2 -1]  value=0  inPortNames=[' '; ' ';]  outPortNames=[' ']  dspbaimage=dspba_prim.svg  text=fprintf('==');  style=Optimised  visibilities=0  advOptions=[]  version=20211007
  Const : DSPBAPrim/Const  primtype=const  nInputs=0  nOutputs=1  omode=Specify via dialog  otype=uint(8)  scale=2^0  rndmethod=Unbiased  factor=1  satmethod=Symmetric  shift_vec=[0 1 2 -1]  value=0  inPortNames=['+'; '+';]  outPortNames=[' ']  dspbaimage=dspba_prim.svg  text=fprintf('%s', num2str(value));  style=Optimised  visibilities=8 + 1024  floatPrecision=float32_m23  warnSaturation=on  version=20211007  SampleTime=inf
  FIFO : DSPBAPrim/FIFO  primtype=fifo  nInputs=3  nOutputs=4  omode=Inherit via internal rule  otype=sfix(16)  scale=2^-15  rndmethod=Unbiased  factor=1  satmethod=Symmetric  shift_vec=[0 1 2 -1]  value=[16 16 16]  inPortNames=['w'; 'd'; 'r'; 'f']  outPortNames=['v'; 'q'; 't'; 'f']  dspbaimage=dspba_prim_tall.svg  text=fprintf('fifo');  style=Optimised  visibilities=263168  version=20211007  user_sclr=off
  FIFO1 : DSPBAPrim/FIFO  primtype=fifo  nInputs=3  nOutputs=4  omode=Inherit via internal rule  otype=sfix(16)  scale=2^-15  rndmethod=Unbiased  factor=1  satmethod=Symmetric  shift_vec=[0 1 2 -1]  value=[16 16 16]  inPortNames=['w'; 'd'; 'r'; 'f']  outPortNames=['v'; 'q'; 't'; 'f']  dspbaimage=dspba_prim_tall.svg  text=fprintf('fifo');  style=Optimised  visibilities=263168  version=20211007  user_sclr=off
  FIFO2 : DSPBAPrim/FIFO  primtype=fifo  nInputs=3  nOutputs=4  omode=Inherit via internal rule  otype=sfix(16)  scale=2^-15  rndmethod=Unbiased  factor=1  satmethod=Symmetric  shift_vec=[0 1 2 -1]  value=[16 16 16]  inPortNames=['w'; 'd'; 'r'; 'f']  outPortNames=['v'; 'q'; 't'; 'f']  dspbaimage=dspba_prim_tall.svg  text=fprintf('fifo');  style=Optimised  visibilities=263168  version=20211007  user_sclr=off
  Goto Tag Visibility : GotoTagVisibility  GotoTag=FFTSize
  Goto Tag Visibility4 : GotoTagVisibility  GotoTag=NSubCarrs
  Rising_edge : $bdroot/Rising_edge
  Rising_edge1 : $bdroot/Rising_edge
  SampleDelay : DSPBAPrim/SampleDelay  Commented=through  primtype=sampdelay  nInputs=1  nOutputs=1  omode=Inherit via internal rule  otype=sfix(16)  scale=2^-15  rndmethod=Unbiased  factor=1  satmethod=Symmetric  shift_vec=[0 1 2 -1]  floatPrecision=float32_m23  value=2  inPortNames=[' '; ' ';]  outPortNames=[' ']  dspbaimage=dspba_prim.svg  text=dpoly(1, eye(1,value+1), 'z')  style=Optimised  visibilities=8 + 1024 + 2^17 + 2^18  flexible=off  slackgroup=0  augmented=0  version=20211007  advOptions=[]
  SampleDelay1 : DSPBAPrim/SampleDelay  Commented=through  primtype=sampdelay  nInputs=1  nOutputs=1  omode=Inherit via internal rule  otype=sfix(16)  scale=2^-15  rndmethod=Unbiased  factor=1  satmethod=Symmetric  shift_vec=[0 1 2 -1]  floatPrecision=float32_m23  value=2  inPortNames=[' '; ' ';]  outPortNames=[' ']  dspbaimage=dspba_prim.svg  text=dpoly(1, eye(1,value+1), 'z')  style=Optimised  visibilities=8 + 1024 + 2^17 + 2^18  flexible=off  slackgroup=0  augmented=0  version=20211007  advOptions=[]
  Scope : Scope  NumInputPorts=4
  Scope1 : Scope  NumInputPorts=4
  SynthesisInfo : DSPBAPrim/SynthesisInfo  primtype=synthinfo  nInputs=0  nOutputs=0  omode=Inherit via internal rule  otype=sfix(16)  scale=2^-15  rndmethod=Truncate  factor=1  satmethod=Symmetric  shift_vec=[0 1 2 -1]  value=99  inPortNames=[' '; ' ';]  outPortNames=[' ']  dspbaimage=dspba_prim_ctrl.jpg  text=fprintf('Style=%s', style);  style=Scheduled  visibilities=2^17+2^18+2^19+2^20+2^21+2^22+2^23+2^24  constraintPair=None  constraintRelation=>  constraintLimit=2  modelRefSign=+  modelRef=''  showSchedule=off  simulationMode=Standard  resetMinimization=Conditional - On for ChannelIn/Out only  version=20220106
  Terminator{1..9} (9 alike) : Terminator
  Transpose : Subsystem  AncestorBlock=DspbAdvFftLibrary/Common/Transpose  Opaque=on  mask(DSP Builder Advanced FFT Blockset){perm=bitrevperm}
      mask prompts: perm "Address permutation"
      mask help: Performs a specialised reordering of a block of data. The size of the block must be a power of 2.
      mask init:
      | N = length(perm);
      | blockSize = 2^N;
      | 
      | % Check parameter legality
      | if ~dspba.check_legal_permutation(perm)
      |     block = gcb;
      |     error('%s: %s is not a legal permutation', ...
      |         block, dspba.perm2str(perm));
      | end
      | 
      | % How many states do we need?
      | allPerms = dspba.calculate_permutation_group(perm);
      | states = size(allPerms,1);
      | 
      | % To avoid reordering the states, we actually need to
      | % generate the addressing using the inverse permutation.
      | inversePerm = allPerms(states,:);
      | 
      | % If states == 1, we need to extend the counter to produce
      | % a dummy state bit to avoid an out-of-range BitExtract.
      | % TransposeAddr will discard the dummy state bit.
      | if 1 < states
      |     counterwidth = N + ceil(log2(states));
      | else
      |     counterwidth = N + 1;
      | end
      mask Help: helpview(dspba.GetHelp('Transpose'));
      mask Display:
      | color('w');
      | image('dspba_fft.jpg');
      | port_label('input',1,'v');
      | port_label('input',2,'d');
      | port_label('output',1,'qv');
      | port_label('output',2,'q');
      | port_label('output',3,'g');
      | text(0.30,0.70,'Transpose');
      | text(0.45,0.55,sprintf('2^{%d}',N),'texmode','on');
      | %text(0.10,0.40,dspba.perm2str(perm));
  channel_BRSC1_in : DSPBAPrim/ChannelIn  primtype=channelin  nInputs=dspba_internal_get_channel_ports(gcb)  nOutputs=dspba_internal_get_channel_ports(gcb)  omode=Inherit via internal rule  otype=sfix(16)  scale=2^-15  rndmethod=Unbiased  factor=1  satmethod=Symmetric  shift_vec=[0 1 2 -1]  value=9  inPortNames=['v'; 'c'; '0'; '1'; '2'; '3'; '4'; '5'; '6'; '7'; '8'; '9'; 'A'; 'B'; 'D'; 'E'; 'F'; 'G'; 'H'; 'I'; 'J'; 'K'; 'L'; 'M'; 'N'; 'O'; 'P'; 'Q'; 'R'; 'S'; 'T'; 'U'; 'W'; 'X'; 'Y'; 'Z']  outPortNames=['v'; 'c'; '0'; '1'; '2'; '3'; '4'; '5'; '6'; '7'; '8'; '9'; 'A'; 'B'; 'D'; 'E'; 'F'; 'G'; 'H'; 'I'; 'J'; 'K'; 'L'; 'M'; 'N'; 'O'; 'P'; 'Q'; 'R'; 'S'; 'T'; 'U'; 'W'; 'X'; 'Y'; 'Z']  dspbaimage=dspba_prim_channel_tall.svg  text=fprintf('In');  style=Optimised  dataSignals=9  foldingEnabled=off  channels=1  sampleRate=200  packetBeginPresent=off  packetBeginEnabled=off  visibilities=dspba_ChannelInVis(gcb)  latencyCorrection=0  scheduleOrigin=on  version=20211214
  channel_BRSC1_out : DSPBAPrim/ChannelOut  primtype=channelout  nInputs=dspba_internal_get_channel_ports(gcb)  nOutputs=dspba_internal_get_channel_ports(gcb)  omode=Inherit via internal rule  otype=sfix(16)  scale=2^-15  rndmethod=Unbiased  factor=1  satmethod=Symmetric  shift_vec=[0 1 2 -1]  value=5  inPortNames=['v'; 'c'; '0'; '1'; '2'; '3'; '4'; '5'; '6'; '7'; '8'; '9']  outPortNames=['v'; 'c'; '0'; '1'; '2'; '3'; '4'; '5'; '6'; '7'; '8'; '9']  dspbaimage=dspba_prim_channel_tall.svg  text=fprintf('Out');  style=Optimised  dataSignals=5  foldingEnabled=off  channels=1  sampleRate=200  packetBeginPresent=off  packetBeginEnabled=off  visibilities=dspba_ChannelOutVis(gcb)  latency=10  latencyCorrection=0  version=20211214
  latch_0L{,1..5} (6 alike) : DSPBAControl/latch_0L
  qv : Outport
  qc : Outport  Port=2
  q : Outport  Port=3
  qsizeout : Outport  Port=4
  time_out : Outport  Port=5
  eAxC_out : Outport  Port=6
  meatadata_sym_out : Outport  Port=7
  tag scope: FFTSize=scoped, NSubCarrs=scoped
  wires:
  SampleDelay1/1 -> latch_0L1/2, [FFTSize]
  SampleDelay/1 -> [NSubCarrs]
  Transpose/3(g) -> latch_0L/1
  Transpose/2(q) -> channel_BRSC1_out/3
  channel_BRSC1_in/5 -> SampleDelay/1
  NSubCarr/1 -> channel_BRSC1_in/5
  channel_BRSC1_in/4 -> SampleDelay1/1
  FFTSize/1 -> channel_BRSC1_in/4
  channel_BRSC1_in/3 -> Transpose/2(d)
  channel_BRSC1_in/2 -> latch_0L/2
  latch_0L/1 -> CmpEQ/2, channel_BRSC1_out/2, Scope1/2
  channel_BRSC1_out/3 -> q/1
  channel_BRSC1_out/2 -> qc/1
  channel_BRSC1_out/1 -> Scope/2, qv/1
  c/1 -> channel_BRSC1_in/2
  v/1 -> channel_BRSC1_in/1
  x/1 -> channel_BRSC1_in/3
  latch_0L1/1 -> channel_BRSC1_out/4, Scope1/4
  channel_BRSC1_out/4 -> qsizeout/1
  time_in/1 -> channel_BRSC1_in/6
  channel_BRSC1_out/5 -> Scope/4, time_out/1
  And/1 -> latch_0L2/1
  CmpEQ/1 -> And/2
  Const/1 -> CmpEQ/1
  latch_0L2/1 -> channel_BRSC1_out/5
  channel_BRSC1_in/7 -> Transpose/3(DC_SC_EN)
  DC_SC_EN/1 -> channel_BRSC1_in/7
  ripple_comp_en/1 -> channel_BRSC1_in/8
  rc_bw_sel/1 -> channel_BRSC1_in/9
  channel_BRSC1_in/8 -> Transpose/4(ripple_comp_en)
  channel_BRSC1_in/9 -> Transpose/5(rc_bw_sel)
  latch_0L5/1 -> latch_0L2/2
  FIFO/3 -> Terminator2/1
  FIFO/4 -> Terminator3/1
  FIFO/1 -> Terminator1/1
  FIFO/2 -> latch_0L3/2
  channel_BRSC1_in/10 -> FIFO/2
  channel_BRSC1_in/11 -> FIFO1/2
  FIFO1/3 -> Terminator5/1
  FIFO1/4 -> Terminator6/1
  FIFO1/1 -> Terminator4/1
  FIFO1/2 -> latch_0L4/2
  Rising_edge1/1 -> latch_0L5/1, FIFO2/3, latch_0L4/1, FIFO1/3, latch_0L3/1, FIFO/3
  channel_BRSC1_in/6 -> FIFO2/2
  FIFO2/3 -> Terminator8/1
  FIFO2/4 -> Terminator9/1
  FIFO2/1 -> Terminator7/1
  Rising_edge/1 -> FIFO2/1, FIFO1/1, FIFO/1
  FIFO2/2 -> latch_0L5/2
  channel_BRSC1_in/1 -> Rising_edge/1, Scope/1, Transpose/1(v)
  Transpose/1(qv) -> And/1, Rising_edge1/1, channel_BRSC1_out/1, Scope1/1, latch_0L1/1
  eAxC/1 -> channel_BRSC1_in/10
  metadata_in/1 -> channel_BRSC1_in/11
  channel_BRSC1_out/6 -> eAxC_out/1
  channel_BRSC1_out/7 -> meatadata_sym_out/1
  latch_0L3/1 -> channel_BRSC1_out/6
  latch_0L4/1 -> channel_BRSC1_out/7
